simulink model "chart_table"  (Simulink 7.9)
settings: Solver=ode45  StartTime=0.0  StopTime=10.0  RelTol=1e-3
values from neighbouring files (symbols this model uses):
  sx_d = [time sx_d]    [WPG_results.m]    (also in WPG_sim.m; control_layer_zmp_com_init.m = [time sx_d_y]; control_layer_zmp_com_init_2.m = [time sx_d_x])
  w = wpg_param.w    [WPG_results.m]    (also in WPG_results_10.m; WPG_results_2.m; WPG_results_3.m; WPG_results_4.m)
  x_d = [time x_d]    [WPG_results.m]    (also in WPG_sim.m; control_layer_zmp_com_init.m = [time x_d_y]; control_layer_zmp_com_init_2.m = [time x_d_x])
settings Model: Creator=pajon  LastModifiedBy=pajon

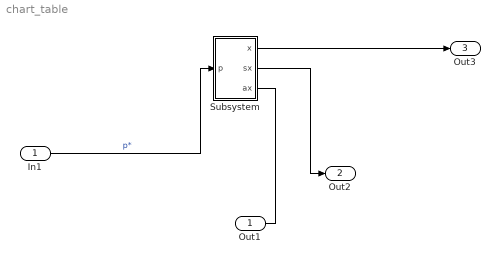
== system chart_table ==
  In1 : Inport
  Subsystem : Subsystem
  Out1 : Outport
  Out2 : Outport  Port=2
  Out3 : Outport  Port=3
  wires:
  In1/1 -> Subsystem/1(p)  "p*"
  Subsystem/1(x) -> Out3/1
  Subsystem/2(sx) -> Out2/1
  Subsystem/3(ax) -> Out1/1

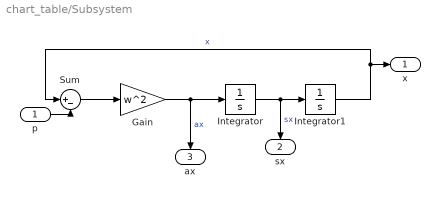
== system chart_table/Subsystem ==
  p : Inport
  Gain : Gain  Gain=w^2
  Integrator : Integrator  InitialCondition=sx_d(1,2)
  Integrator1 : Integrator  InitialCondition=x_d(1,2)
  Sum : Sum  Inputs=|+-
  x : Outport
  sx : Outport  Port=2
  ax : Outport  Port=3
  wires:
  Integrator/1 -> Integrator1/1, sx/1  "sx"
  Integrator1/1 -> Sum/1, x/1  "x"
  Gain/1 -> Integrator/1, ax/1  "ax"
  Sum/1 -> Gain/1
  p/1 -> Sum/2
